simulink model "MODBUS_TCP_Test"  (R2024a)
settings: Solver=FixedStepAuto  StartTime=0.0  StopTime=10.0  RelTol=1e-3  EnableMultiTasking=on
libraries: px4Utilslib x1
settings Model: ExtModeTrigDuration=10  Creator=root  LastModifiedBy=root
settings SolverCC: PositivePriorityOrder=on
settings OptimizationCC: OptimizeBlockIOStorage=off  BufferReuse=off  ReuseModelBlockBuffer=off  GlobalBufferReuse=off  ExpressionFolding=off  EnableMemcpy=off  PassReuseOutputArgsAs=Individual arguments  LocalBlockOutputs=off  ZeroExternalMemoryAtStartup=off  ZeroInternalMemoryAtStartup=off  MaxStackSize=64  OptimizeDataStoreBuffers=off  BusAssignmentInplaceUpdate=off  OptimizationLevel=level0  OptimizationCustomize=off  EfficientTunableParamExpr=on
settings DebuggingCC: ParameterTunabilityLossMsg=error
settings HardwareCC: ProdBitPerPointer=32  ProdBitPerSizeT=32  ProdBitPerPtrDiffT=32  ProdLargestAtomicInteger=Long  ProdLargestAtomicFloat=Double  ProdWordSize=32  ProdLongLongMode=on  ProdHWDeviceType=ARM Compatible->ARM Cortex
settings SFSimCC: SimUserSources=modbus_tcp_client.cpp  SimUserIncludeDirs=/home/judson/Desktop/Pixhawk/MATLAB/MODBUS_TCP_Test  MATLABDynamicMemAlloc=off  CustomCodeGlobalsAsFunctionIO=on  SimTargetLang=C++
settings SFSimCC: SimCustomHeaderCode=|
  | #include <netinet/in.h>
  | #include <sys/types.h>
  | #include <sys/socket.h>
  | #include <arpa/inet.h>
  | #include <errno.h>
  | #include <stdio.h>
  | #include <string.h>
  | #include <unistd.h>
  | #include "modbus_tcp_client.h"
settings RTWCC: Description=Embedded Coder  SystemTargetFile=ert.tlc  HardwareBoard=PX4 Pixhawk 6x  TLCOptions="-aInlineSetEventsForThisBaseRateFcn=TLC_FALSE -aSuppressMultiTaskScheduler=TLC_FALSE  -aRateBasedStepFcn=0"  TemplateMakefile=ert_default_tmf  RTWUseSimCustomCode=on  CustomInclude=/home/judson/Desktop/Pixhawk/MATLAB/MODBUS_TCP_Test  CustomSource=modbus_tcp_client.cpp  Toolchain=GNU Tools for PX4 Autopilots  BuildConfiguration=Debug  TargetLang=C++
settings RTWCC: CustomHeaderCode=|
  | #include <netinet/in.h>
  | #include <sys/types.h>
  | #include <sys/socket.h>
  | #include <arpa/inet.h>
  | #include <errno.h>
  | #include <stdio.h>
  | #include <string.h>
  | #include <unistd.h>
  | #include "modbus_tcp_client.h"
settings CodeAppCC: ForceParamTrailComments=on  IgnoreCustomStorageClasses=off  OperatorAnnotations=on  SimulinkDataObjDesc=on  SFDataObjDesc=on  MATLABFcnDesc=on  InsertBlockDesc=on  EnableCustomComments=on  ReqsInCode=on
settings ERTTargetCC: TargetLangStandard=C++11 (ISO)  SupportNonFinite=off  ExtModeTransport=3  ExtModeStaticAlloc=on  ExtModeStaticAllocSize=1024  ExtModeMexFile=ext_xcp  ExtModeIntrfLevel=Level2 - Open  PreserveIfCondition=on

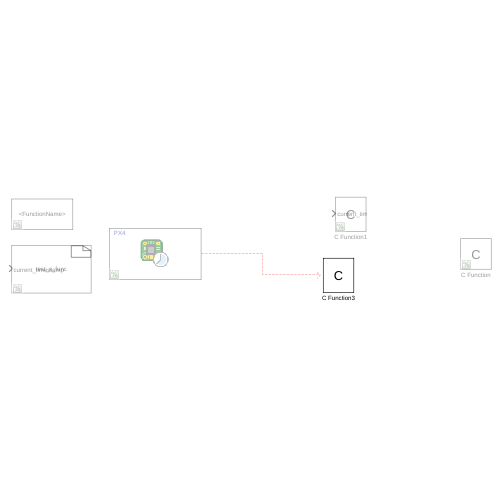
[thumbnail: Simulink's stored preview of the top-level diagram]
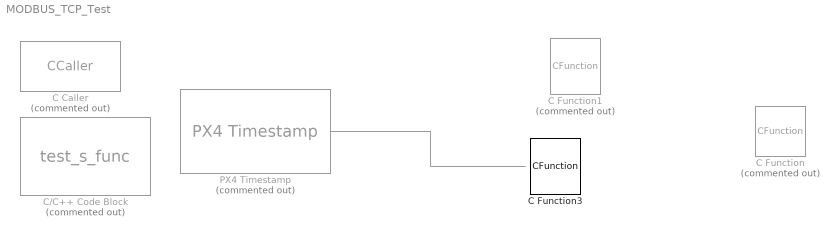
== system MODBUS_TCP_Test ==
  C Caller : CCaller  Commented=on
  C Function : CFunction  Commented=on  OutputCode=|  CodegenOutputCode=|  SampleTime=0.7
      OutputCode=|
      | int sock = socket(AF_INET, SOCK_DGRAM, 0);
      | 
      | struct sockaddr_in server_addr;
      | memset(&server_addr, 0, sizeof(server_addr));
      | server_addr.sin_family = AF_INET;
      | server_addr.sin_port = htons(8080);
      | 
      | if (inet_pton(AF_INET, "192.168.0.210", &server_addr.sin_addr) <= 0) {
      |   close(sock);
      | }
      | 
      | 
      | int result = connect(sock, (struct sockaddr*)&server_addr, sizeof(server_addr));
      | if (result < 0) {
      |   close(sock);
      | }
      | 
      | char message[] = "Hello from PX4 very fast!";
      | send(sock, message, strlen(message), 0);
      | 
      | close(sock);
      CodegenOutputCode=|
      | int sock = socket(AF_INET, SOCK_DGRAM, 0);
      | 
      | struct sockaddr_in server_addr;
      | memset(&server_addr, 0, sizeof(server_addr));
      | server_addr.sin_family = AF_INET;
      | server_addr.sin_port = htons(8080);
      | 
      | if (inet_pton(AF_INET, "192.168.0.210", &server_addr.sin_addr) <= 0) {
      |   close(sock);
      | }
      | 
      | 
      | int result = connect(sock, (struct sockaddr*)&server_addr, sizeof(server_addr));
      | if (result < 0) {
      |   close(sock);
      | }
      | 
      | char message[] = "Hello from PX4 very fast!";
      | send(sock, message, strlen(message), 0);
      | 
      | close(sock);
  C Function1 : CFunction  Commented=on  OutputCode=|  CodegenOutputCode=|  SimCustomHeaderFile="#include \"modbus_tcp_client.h\""  CustomHeaderFile="#include \"modbus_tcp_client.h\""
      OutputCode=|
      | static ModbusTCPClient modbus("192.168.0.129", 5020);
      |     modbus.setTimeout(100);
      | 
      |     if (!modbus.connectServer()) {
      |         printf("Failed to connect to MODBUS server!\n");
      |         return 1;
      |     }
      | 
      |     uint16_t registerValues[3] = {100, 200, 300};
      |     ModbusError result = modbus.writeMultipleHoldingRegisters(1, 3, registerValues);
      | 
      |     if (result == ModbusError::NONE) {
      |         printf("Successfully wrote multiple Holding Registers!\n");
      |     } else {
      |         printf("Error writing multiple Holding Registers: %d\n", static_cast<int>(result));
      |     }
      |     
      |     uint16_t registerValues2[3] = {700, 600, 500};
      |     ModbusError result2 = modbus.writeMultipleHoldingRegisters(6, 3, registerValues2);
      | 
      |     if (result2 == ModbusError::NONE) {
      |         printf("Successfully wrote multiple Holding Registers!\n");
      |     } else {
      |         printf("Error writing multiple Holding Registers: %d\n", static_cast<int>(result2));
      |     }
      CodegenOutputCode=|
      | static ModbusTCPClient modbus("192.168.0.129", 5020);
      |     modbus.setTimeout(100);
      | 
      |     if (!modbus.connectServer()) {
      |         printf("Failed to connect to MODBUS server!\n");
      |         return 1;
      |     }
      | 
      |     uint16_t registerValues[3] = {100, 200, 300};
      |     ModbusError result = modbus.writeMultipleHoldingRegisters(1, 3, registerValues);
      | 
      |     if (result == ModbusError::NONE) {
      |         printf("Successfully wrote multiple Holding Registers!\n");
      |     } else {
      |         printf("Error writing multiple Holding Registers: %d\n", static_cast<int>(result));
      |     }
      |     
      |     uint16_t registerValues2[3] = {700, 600, 500};
      |     ModbusError result2 = modbus.writeMultipleHoldingRegisters(6, 3, registerValues2);
      | 
      |     if (result2 == ModbusError::NONE) {
      |         printf("Successfully wrote multiple Holding Registers!\n");
      |     } else {
      |         printf("Error writing multiple Holding Registers: %d\n", static_cast<int>(result2));
      |     }
  C Function3 : CFunction  OutputCode=|  CodegenOutputCode=|  SampleTime=10  SimCustomHeaderFile="#include \"modbus_tcp_client.h\""  SimCustomSourceFile=""  CustomHeaderFile="#include \"modbus_tcp_client.h\""  CustomSourceFile=""
      OutputCode=|
      | static ModbusTCPClient modbus("192.168.0.129", 5020, 10, 10, 10, 10);
      | 
      | if (!modbus.isConnected()) {  // Only connect if not already connected
      |     modbus.setTimeout(1000);
      |     if (!modbus.connectServer()) {
      |         printf("Failed to connect to MODBUS server!\n");
      |         return 1;
      |     }
      | }
      | 
      | 
      | // Read fresh MODBUS values
      | modbus.readAll();
      | 
      | uint16_t new_value = modbus.getHoldingRegister(0);
      | printf("After readAll: Holding Register: %u\n", new_value);
      CodegenOutputCode=|
      | static ModbusTCPClient modbus("192.168.0.129", 5020, 10, 10, 10, 10);
      | 
      | if (!modbus.isConnected()) {  // Only connect if not already connected
      |     modbus.setTimeout(1000);
      |     if (!modbus.connectServer()) {
      |         printf("Failed to connect to MODBUS server!\n");
      |         return 1;
      |     }
      | }
      | 
      | 
      | // Read fresh MODBUS values
      | modbus.readAll();
      | 
      | uint16_t new_value = modbus.getHoldingRegister(0);
      | printf("After readAll: Holding Register: %u\n", new_value);
  C/C++ Code Block : S-Function  Commented=on  FunctionName=test_s_func  SFunctionModules=test_s_func_wrapper.cpp  SFunctionDeploymentMode=off  EnableBusSupport=off  mask(S-Function Builder){}
      mask help: Simulink:masks:SFunctionBuilder_MD
      mask init:
      | val = [[.9  0.75 0.75 1 1 .9 .9 1]',[1 1 0.75 0.75 .9 .9 1 .9]'];try , sys = get_param(gcb,'SfunBuilderFcnName');if isempty(sys), sys = get_param(gcb,'FunctionName'); end,catch, sys = get_param(gcb,'FunctionName'); end
      settings: CopyFcn=set_param(gcbh,'LinkStatus','none')  OpenFcn=sfunctionwizard(gcbh)
      mask Display:
      | plot(val(:,1),val(:,2))
      | disp(sys)
      | port_label('input',1,sprintf('%s', 'current\_timestamp'),'interpreter','tex')
  PX4 Timestamp : px4Utilslib/PX4 Timestamp  Commented=on  SampleTime=10
      settings: SourceProductName=PX4 Utility Blocks
  wires:
  PX4 Timestamp/1 -> ?
